simulink model "Expt_4"  (R2016a)
settings: Solver=VariableStepAuto  StartTime=0.0  StopTime=10.0  RelTol=1e-3
PreLoadFcn:
  | bitRate=500000;
  | bitsPerFrame=200;
  | maxDopplerShift=200;
  | delayVector=[0:3]*(4e-6);
  | gainVector=[0:3]*(-3);
  | LOSDopplerShift=100;
  | KFactor=10;
libraries: commchan3 x2, commrandsrc3 x1, commdigbbndpm3 x1
CloseFcn:
  | clear bitRate
  | clear bitsPerFrame
  | clear maxDopplerShift
  | clear delayVector
  | clear gainVector
  | clear LOSDopplerShift
  | clear KFactor
settings Model: Creator=viren  LastModifiedBy=viren

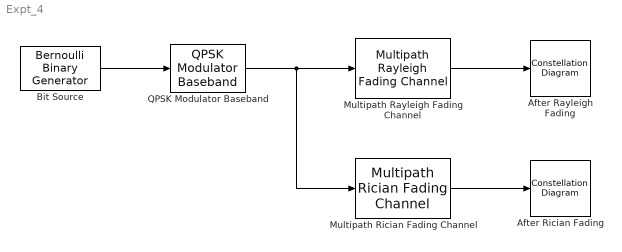
== system Expt_4 ==
  After Rayleigh Fading : ConstellationDiagram
  After Rician Fading : ConstellationDiagram
  Bit Source : commrandsrc3/Bernoulli Binary Generator  ProbabilityOfZero=0.5  SeedSource=Auto  Seed=0  SampleTime=1  SamplesPerFrame=1  OutputDataType=boolean  SimulateUsing=Interpreted execution
  Multipath Rayleigh Fading Channel : commchan3/Multipath Rayleigh Fading Channel  maxDopplerShift=maxDopplerShift  spectrumType=Jakes  sigmaGaussian=1/sqrt(2)  coeffRounded=[1 -1.72 0.785]  freqMinMaxRJakes=[0 1]  freqMinMaxAJakes=[0 1]  sigmaGaussian1=1/sqrt(2)  sigmaGaussian2=1/sqrt(2)  centerFreqGaussian1=0.0  centerFreqGaussian2=0.0  gainGaussian1=0.5  gainGaussian2=0.5  coeffBell=9  dopplerSpectrum=doppler.jakes  pathDelays=delayVector  avgPathGaindB=gainVector  normalizePathGains=on  seed=12345  enableProbe=0  openVisAtStart=on  outPathGains=off  outDelay=off
  Multipath Rician Fading Channel : commchan3/Multipath Rician Fading Channel  K=KFactor  fdLOS=LOSDopplerShift  thetaLOS=0  maxDopplerShift=maxDopplerShift  spectrumType=Jakes  sigmaGaussian=1/sqrt(2)  coeffRounded=[1 -1.72 0.785]  freqMinMaxRJakes=[0 1]  freqMinMaxAJakes=[0 1]  sigmaGaussian1=1/sqrt(2)  sigmaGaussian2=1/sqrt(2)  centerFreqGaussian1=0  centerFreqGaussian2=0  gainGaussian1=0.5  gainGaussian2=0.5  coeffBell=9  dopplerSpectrum=doppler.jakes  pathDelays=delayVector  avgPathGaindB=gainVector  normalizePathGains=on  seed=12345  enableProbe=0  openVisAtStart=on  outPathGains=off  outDelay=off
  QPSK Modulator Baseband : commdigbbndpm3/QPSK Modulator Baseband  InType=Bit  Enc=Gray  Ph=pi/4  outDtype=double  outWordLen=16  outUDDataType=sfix(16)  outFracLenMode=Best precision  outFracLen=15  outDataTypeStr=double  outLastDataTypeStr=double
  wires:
  Bit Source/1 -> QPSK Modulator Baseband/1
  QPSK Modulator Baseband/1 -> Multipath Rician Fading Channel/1, Multipath Rayleigh Fading Channel/1
  Multipath Rayleigh Fading Channel/1 -> After Rayleigh Fading/1
  Multipath Rician Fading Channel/1 -> After Rician Fading/1
